simulink model "SAME5xPIM_MCLV2_MotorControl"  (R2021a)
settings: Solver=FixedStepDiscrete  StartTime=0.0  StopTime=10.0  FixedStep=5e-5  RelTol=1e-3  EnableMultiTasking=on
InitFcn:
  | % DC Voltage
  | VDC = 24;
  | 
  | % Intersective PMW
  | Vmax = VDC/2;
  | Imax = 4;
  | 
  | Ts = 1e-4;
  | 
  | 
  | % pole paires
  | p = 4;
  | 
  | % QEI
  | lines = 4*1000;
  | eleclines = lines/p;
  | inveleclines = 1/eleclines
  | gainQEIspeed = 2*pi/Ts/lines
  | 
  | % Electrical parameters
  | R=0.656; L=0.35e-3; Phif=0.0066;
  | % Mechanical parameters
  | F=1.e-05; J=1e-05; C0 = 0.01;%10;%1;
undefined symbols (not defined in the file): B27, PA08, PA09, PA10, PA11, PA12, PA13, PA16, PA17, PA18, pad0, pad1, pad2, pad3, PC16, PC17, PC18, Pin, SAME54P20A, Timer, TQFP128, wo0, wo1, wo2, wo4, wo5, wo6
libraries: MCHP_Blockset x10, simulink x8, dsparch4 x1
(part 2 of 2)

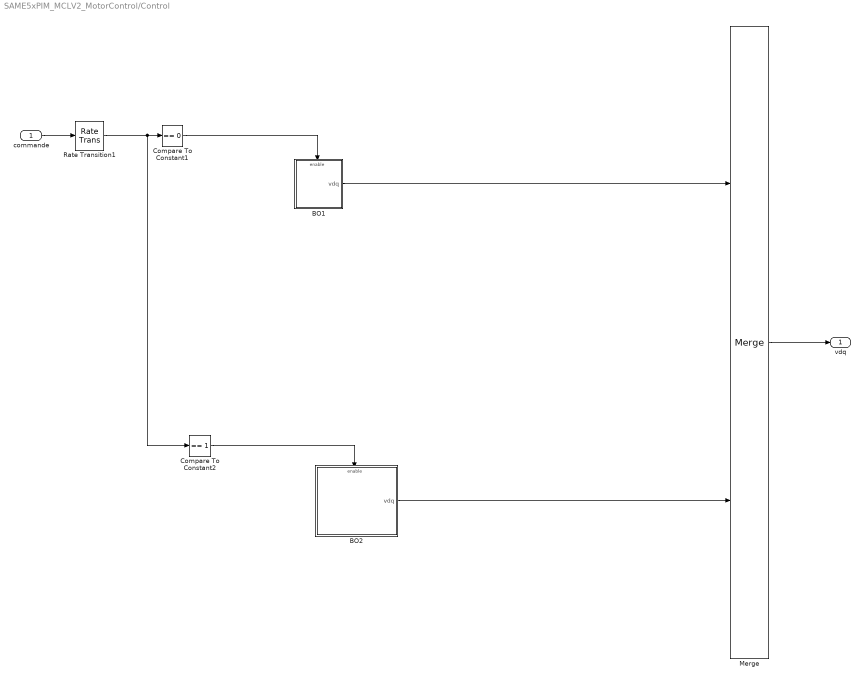
== system SAME5xPIM_MCLV2_MotorControl/Control ==
  commande : Inport
  BO1 : Subsystem
  BO2 : Subsystem
  Compare To Constant1 : simulink/Logic and Bit Operations/Compare To Constant  relop===  const=0  OutDataTypeStr=boolean
  Compare To Constant2 : simulink/Logic and Bit Operations/Compare To Constant  relop===  const=1  OutDataTypeStr=boolean
  Merge : Merge
  Rate Transition1 : RateTransition
  vdq : Outport  VectorParamsAs1DForOutWhenUnconnected=off
  wires:
  Rate Transition1/1 -> Compare To Constant1/1, Compare To Constant2/1
  Compare To Constant1/1 -> BO1/Enable
  commande/1 -> Rate Transition1/1
  Merge/1 -> vdq/1
  Compare To Constant2/1 -> BO2/Enable
  BO1/1(vdq) -> Merge/1
  BO2/1(vdq) -> Merge/2

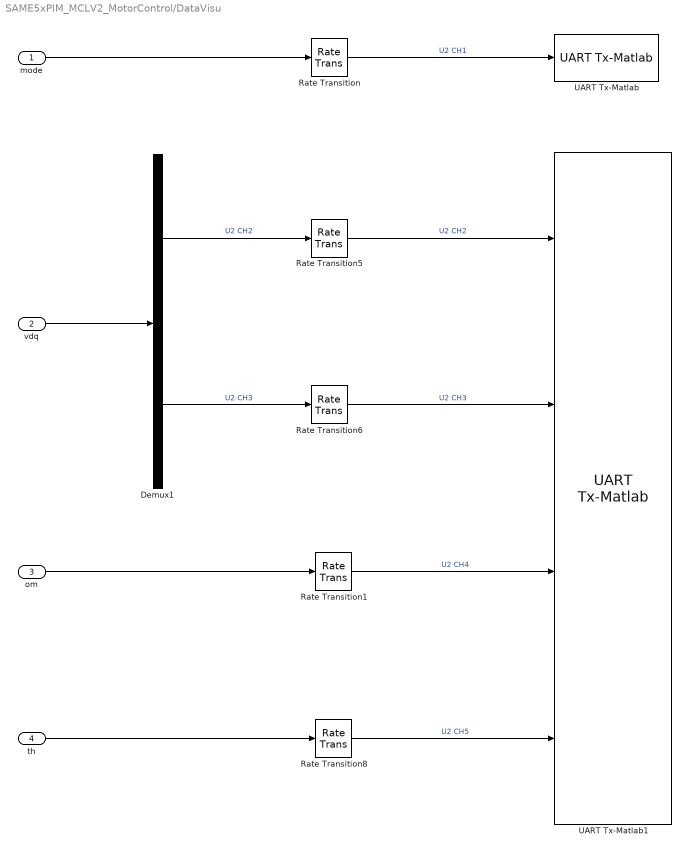
== system SAME5xPIM_MCLV2_MotorControl/DataVisu ==
  mode : Inport
  vdq : Inport  Port=2
  om : Inport  Port=3
  th : Inport  Port=4
  Demux1 : Demux  Outputs=2
  Rate Transition{,1,5..6,8} (5 alike) : RateTransition
  UART Tx-Matlab : MCHP_Blockset/BUS UART/UART Tx-Matlab  UART_REF=2  CHANNELS=[1]  AllOrNothing=off  SampleTime=.1  MCHP_MASTERLINK=SAME5xPIM_MCLV2_MotorControl/Microchip Master  MCHP_COMPILED_INFO="CompiledSampleTime= [0.10000000000000000555   0 ];CompiledInportDataTypes=[  5 ];CompiledInportDataWidth=[1];"
      settings: SourceProductName=MPLAB Device Blocks for Simulink
  UART Tx-Matlab1 : MCHP_Blockset/BUS UART/UART Tx-Matlab  UART_REF=2  CHANNELS=[2:5]  AllOrNothing=off  SampleTime=0.0005  MCHP_MASTERLINK=SAME5xPIM_MCLV2_MotorControl/Microchip Master  MCHP_COMPILED_INFO="CompiledSampleTime= [0.00050000000000000001041   0 ];CompiledInportDataTypes=[  1   1   1   1 ];CompiledInportDataWidth=[1  1  1  1];"
      settings: SourceProductName=MPLAB Device Blocks for Simulink
  wires:
  vdq/1 -> Demux1/1
  th/1 -> Rate Transition8/1
  Rate Transition5/1 -> UART Tx-Matlab1/1  "U2 CH2"
  Rate Transition8/1 -> UART Tx-Matlab1/4  "U2 CH5"
  Rate Transition1/1 -> UART Tx-Matlab1/3  "U2 CH4"
  Demux1/2 -> Rate Transition6/1  "U2 CH3"
  Rate Transition6/1 -> UART Tx-Matlab1/2  "U2 CH3"
  Demux1/1 -> Rate Transition5/1  "U2 CH2"
  om/1 -> Rate Transition1/1
  Rate Transition/1 -> UART Tx-Matlab/1  "U2 CH1"
  mode/1 -> Rate Transition/1

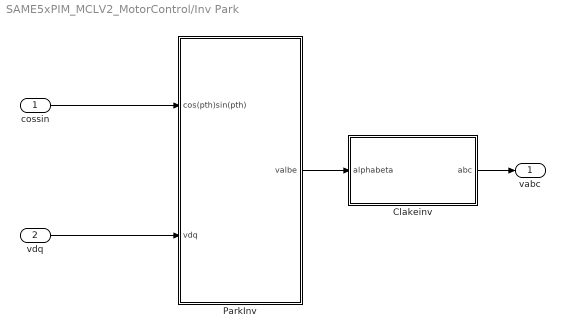
== system SAME5xPIM_MCLV2_MotorControl/Inv Park ==
  cossin : Inport
  vdq : Inport  Port=2  PortDimensions=2
  Clakeinv : Subsystem
  ParkInv : Subsystem
  vabc : Outport  VectorParamsAs1DForOutWhenUnconnected=off
  wires:
  vdq/1 -> ParkInv/2(vdq)
  cossin/1 -> ParkInv/1(cos(pth)sin(pth))
  ParkInv/1(valbe) -> Clakeinv/1(alphabeta)
  Clakeinv/1(abc) -> vabc/1

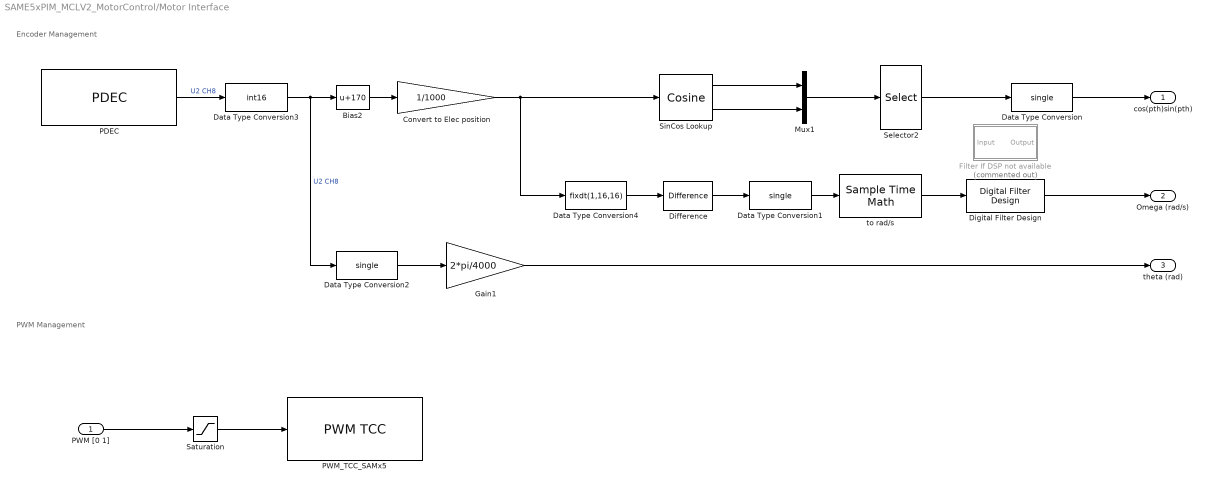
== system SAME5xPIM_MCLV2_MotorControl/Motor Interface ==
  note: Encoder Management
  note: PWM Management
  PWM [0 1] : Inport
  Bias2 : Bias  Bias=170
  Convert to Elec position : Gain  Gain=1/1000  OutDataTypeStr=fixdt(0,16,16)
  Data Type Conversion : DataTypeConversion  OutDataTypeStr=single
  Data Type Conversion1 : DataTypeConversion  OutDataTypeStr=single
  Data Type Conversion2 : DataTypeConversion  OutDataTypeStr=single
  Data Type Conversion3 : DataTypeConversion  OutDataTypeStr=int16  ConvertRealWorld=Stored Integer (SI)
  Data Type Conversion4 : DataTypeConversion  OutDataTypeStr=fixdt(1,16,16)  ConvertRealWorld=Stored Integer (SI)
  Difference : simulink/Discrete/Difference  ICPrevInput=0  OutMin=[]  OutMax=[]  OutDataType=fixdt(1, 16)  OutScaling=2^-10  DoSatur=off
  Digital Filter Design : dsparch4/Digital Filter Design  mwdsp_browser_bugfix_var=off
  Filter If DSP not available : Subsystem  Tag=FilterWizardSubSystem  Commented=on
      settings: ErrorFcn=dspFilterRealizedInBasicElemsAlgLoopErrFcnCallback
  Gain1 : Gain  Gain=2*pi/4000
  Mux1 : Mux  Inputs=2
  PDEC : MCHP_Blockset/QEI/PDEC  Mode=Quadrature Encoder  index=Reset counter  QDI0=PC16 / Pin[70]  QDI0_txt=Dynamic Options  QDI1=PC17 / Pin[71]  QDI1_txt=Dynamic Options  QDI2=PC18 / Pin[72]  QDI2_txt=Dynamic Options  maxCounterReset=-1  AutoCorrection=off  AutoCorrection_override=on  info=0  MCHP_MASTERLINK=SAME5xPIM_MCLV2_MotorControl/Microchip Master  SampleTime=1e-4  MCHP_PORT={PDEC A}{PDEC_QDI0}5:0:P80;{PDEC B}{PDEC_QDI1}5:0:P81;{PDEC index}{PDEC_QDI2}5:0:P82;  MAXPOS_INPUT=off  RESET_INPUT=off  OutputCounter=on  OutputCounter_Signed=unsigned  OutputRevolution=off  CounterRevolution_length=Counter is 13 bits ; revolution is 3 bits  OutputRevolution_Signed=unsigned  FILTER="250 (ns)  ->  freq 2 (MHz)"  FILTER_TXT="250 (ns)  ->  freq 2 (MHz)"  SWAP=off  QDI_invert_0=off  QDI_invert_1=off  QDI_invert_2=off
      settings: SourceProductName=MPLAB Device Blocks for Simulink
  PWM_TCC_SAMx5 : MCHP_Blockset/PWM IO/PWM TCC  TCCREF=TCC 0  WAVE_choice=Center aligned PWM  MaxPeriod_s=5e-5  OTMX=Default  WO0=Dynamic Options  WO0_TXT=PA08 / Pin[33] / wo0  WO1=Dynamic Options  WO1_TXT=PA09 / Pin[34] / wo1  WO2=Dynamic Options  WO2_TXT=PA10 / Pin[35] / wo2  WO3=Dynamic Options  WO3_TXT=Not Used  WO4=Dynamic Options  WO4_TXT=PA16 / Pin[66] / wo4  WO5=Dynamic Options  WO5_TXT=PA17 / Pin[67] / wo5  WO6=Dynamic Options  WO6_TXT=PA18 / Pin[68] / wo6  WO7=Dynamic Options  WO7_TXT=Not Used  info=0  evalin_ws=PWM0max=MCHP_Fun.Hex2num('40A3860000000000');PWM0max=MCHP_Fun.Hex2num('40A3860000000000');PWM0max=MCHP_Fun.Hex2num('40A3860000000000');  SampleTime=1e-4  MCHP_PORT={PWM0_H0}{TCC0_WO0}5:1:P8;{PWM0_H1}{TCC0_WO1}5:1:P9;{PWM0_H2}{TCC0_WO2}5:1:P10;{PWM0_L0}{TCC0_WO4}5:1:P16;{PWM0_L1}{TCC0_WO5}5:1:P17;{PWM0_L2}{TCC0_WO6}5:1:P18;  MCHP_MASTERLINK=SAME5xPIM_MCLV2_MotorControl/Microchip Master  INVEN_WO0=off  INVEN_WO1=off  INVEN_WO2=off  INVEN_WO3=off  INVEN_WO4=off  INVEN_WO5=off  INVEN_WO6=off  INVEN_WO7=off  SWAP_PWM0=off  SWAP_PWM1=off  SWAP_PWM2=off  SWAP_PWM3=off  POL_PWM0=off  POL_PWM1=off  POL_PWM2=off  POL_PWM3=off  POL_PWM4=off  POL_PWM5=off  InitPeriod_s=5e-5  InitDutyCycle_s=2.5e-5  InitDeadTimeH_s=0.5e-6  InitDeadTimeL_s=0.5e-6  InitOutputOverride=0  InitOutputOverride_val=0  BlockInput_VectorScalar=Vectors (grouped by function)  BlockInput_Period=Not a block input  BlockInput_DutyCycle=a Floating Point input within range [0 1]  BlockInput_DeadTime=Not a block input  BlockInput_OutputOverride=Not a block input
      settings: SourceProductName=MPLAB Device Blocks for Simulink
  Saturation : Saturate  UpperLimit=0.98  LowerLimit=0.02  LinearizeAsGain=off  OutDataTypeStr=double
  Selector2 : Selector  InputPortWidth=2  IndexOptions=Index vector (dialog)  Indices=[2 1]  OutputSizes=1
  SinCos Lookup : simulink/Lookup Tables/Cosine  Formula=sin(2*pi*u) and cos(2*pi*u)  NumDataPoints=(2^12)+1  OutputWordLength=16  InternalRulePriority=Precision
      settings: SourceProductBaseCode=SL
  to rad/s : SampleTimeMath  TsampMathOp=/  weightValue=(4)/(2*pi)
  cos(pth)sin(pth) : Outport  VectorParamsAs1DForOutWhenUnconnected=off
  Omega (rad/s) : Outport  Port=2  PortDimensions=1  VectorParamsAs1DForOutWhenUnconnected=off
  theta (rad) : Outport  Port=3  VectorParamsAs1DForOutWhenUnconnected=off
  wires:
  Saturation/1 -> PWM_TCC_SAMx5/1
  PWM [0 1]/1 -> Saturation/1
  Convert to Elec position/1 -> Data Type Conversion4/1, SinCos Lookup/1
  to rad/s/1 -> Digital Filter Design/1
  Bias2/1 -> Convert to Elec position/1
  PDEC/1 -> Data Type Conversion3/1  "U2 CH8"
  Digital Filter Design/1 -> Omega (rad/s)/1
  Data Type Conversion/1 -> cos(pth)sin(pth)/1
  Mux1/1 -> Selector2/1
  Selector2/1 -> Data Type Conversion/1
  SinCos Lookup/2 -> Mux1/2
  SinCos Lookup/1 -> Mux1/1
  Data Type Conversion3/1 -> Data Type Conversion2/1, Bias2/1  "U2 CH8"
  Data Type Conversion2/1 -> Gain1/1
  Gain1/1 -> theta (rad)/1
  Difference/1 -> Data Type Conversion1/1
  Data Type Conversion4/1 -> Difference/1
  Data Type Conversion1/1 -> to rad/s/1

== system SAME5xPIM_MCLV2_MotorControl/PWM ==
  vabc : Inport
  50% average duty-cycle : Bias  Bias=0.5
  Gain : Gain  Gain=1/VDC  OutDataTypeStr=double
  PWM [0 1] : Outport  VectorParamsAs1DForOutWhenUnconnected=off
  wires:
  vabc/1 -> Gain/1
  50% average duty-cycle/1 -> PWM [0 1]/1
  Gain/1 -> 50% average duty-cycle/1

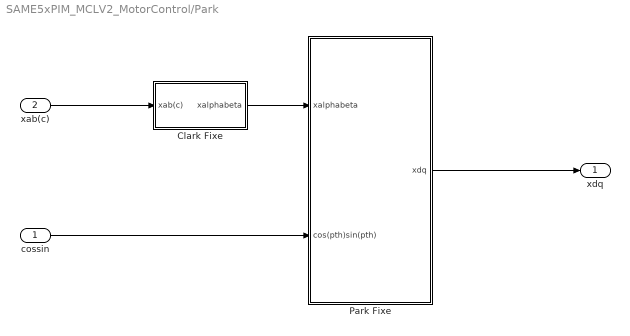
== system SAME5xPIM_MCLV2_MotorControl/Park  ==
  cossin : Inport
  xab(c) : Inport  Port=2
  Clark Fixe : Subsystem
  Park Fixe : Subsystem
  xdq : Outport  VectorParamsAs1DForOutWhenUnconnected=off
  wires:
  Clark Fixe/1(xalphabeta) -> Park Fixe/1(xalphabeta)
  xab(c)/1 -> Clark Fixe/1(xab(c))
  cossin/1 -> Park Fixe/2(cos(pth)sin(pth))
  Park Fixe/1(xdq) -> xdq/1

== system SAME5xPIM_MCLV2_MotorControl/Selector ==
  BTN_S2 : MCHP_Blockset/Digital IO/Digital Input  PORT=Dynamic Options  PORT_TXT="D   [ 0  1  8  9  10  11  12  20  21 ]"  PIN=9  PACK=off  SIMULTANEOUS=off  ORDERING=None  SampleTime=.1  MCHP_PORT={Digital In}{DIN}2:0:D9;  MCHP_MASTERLINK=SAME5xPIM_MCLV2_MotorControl/Microchip Master
      settings: SourceProductName=MPLAB Device Blocks for Simulink
  Toggle (4 states)1 : Subsystem
  Mode : Outport  VectorParamsAs1DForOutWhenUnconnected=off
  tag scope: mode=global
  wires:
  BTN_S2/1 -> Toggle (4 states)1/1(In1)
  Toggle (4 states)1/1(Mode) -> [mode], Mode/1

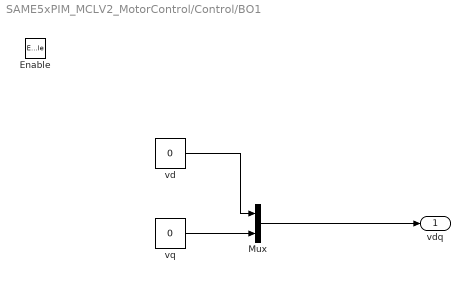
== system SAME5xPIM_MCLV2_MotorControl/Control/BO1 ==
  Enable : EnablePort
  Mux : Mux  Inputs=2
  vd : Constant  Value=0  OutMin=[-12]  OutMax=[12]  OutDataTypeStr=single
  vq : Constant  Value=0  OutMin=[-12]  OutMax=[12]  OutDataTypeStr=single
  vdq : Outport  VectorParamsAs1DForOutWhenUnconnected=off
  wires:
  vd/1 -> Mux/1
  Mux/1 -> vdq/1
  vq/1 -> Mux/2

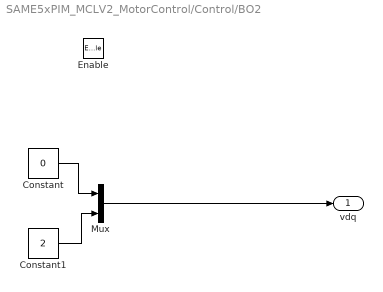
== system SAME5xPIM_MCLV2_MotorControl/Control/BO2 ==
  Enable : EnablePort
  Constant : Constant  Value=0  OutDataTypeStr=single
  Constant1 : Constant  Value=2  OutDataTypeStr=single
  Mux : Mux  Inputs=2
  vdq : Outport  VectorParamsAs1DForOutWhenUnconnected=off
  wires:
  Constant1/1 -> Mux/2
  Constant/1 -> Mux/1
  Mux/1 -> vdq/1

== system SAME5xPIM_MCLV2_MotorControl/Inv Park/Clakeinv ==
  alphabeta : Inport
  Clarke1 : Product  Multiplication=Matrix(*)  RndMeth=Simplest  OutDataTypeStr=Inherit: Same as first input
  Constant Magnitude : Constant  Value=[1 0 ; -1/2 sqrt(3)/2 ;-1/2 -sqrt(3)/2]'  OutDataTypeStr=Inherit: Inherit via back propagation  SampleTime=-1
  Math Function : Math  Operator=transpose  SignedPower=on  SaturateOnIntegerOverflow=on
  abc : Outport  VectorParamsAs1DForOutWhenUnconnected=off
  wires:
  alphabeta/1 -> Math Function/1
  Constant Magnitude/1 -> Clarke1/2
  Math Function/1 -> Clarke1/1
  Clarke1/1 -> abc/1

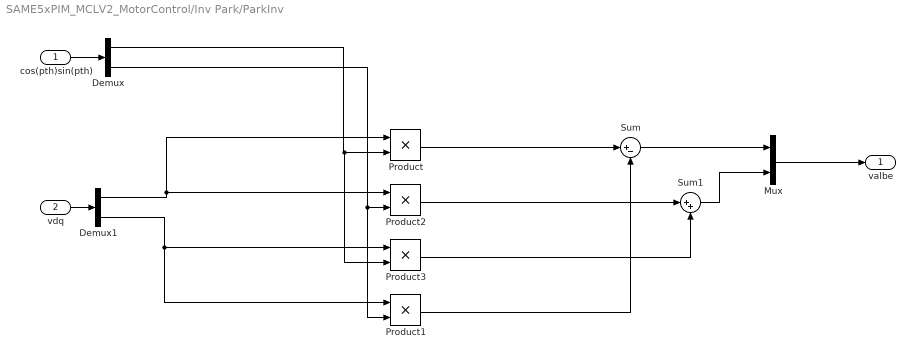
== system SAME5xPIM_MCLV2_MotorControl/Inv Park/ParkInv ==
  cos(pth)sin(pth) : Inport
  vdq : Inport  Port=2
  Demux : Demux  Outputs=2
  Demux1 : Demux  Outputs=2
  Mux : Mux  Inputs=2
  Product{,1..3} (4 alike) : Product
  Sum : Sum  Inputs=|+-
  Sum1 : Sum  Inputs=|++
  valbe : Outport  VectorParamsAs1DForOutWhenUnconnected=off
  wires:
  vdq/1 -> Demux1/1
  cos(pth)sin(pth)/1 -> Demux/1
  Sum/1 -> Mux/1
  Demux1/1 -> Product2/1, Product/1
  Demux1/2 -> Product3/1, Product1/1
  Sum1/1 -> Mux/2
  Product1/1 -> Sum/2
  Product/1 -> Sum/1
  Demux/1 -> Product3/2, Product/2
  Demux/2 -> Product2/2, Product1/2
  Mux/1 -> valbe/1
  Product2/1 -> Sum1/1
  Product3/1 -> Sum1/2

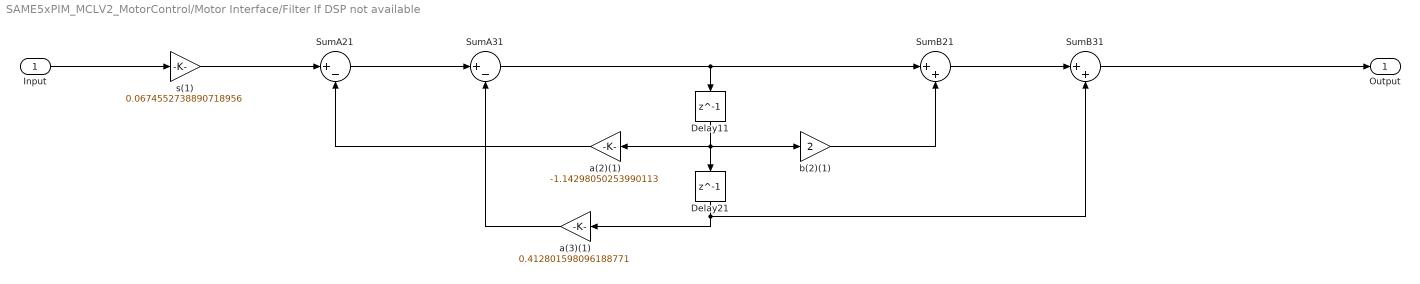
== system SAME5xPIM_MCLV2_MotorControl/Motor Interface/Filter If DSP not available ==
  Input : Inport
  Delay11 : Delay  DelayLength=1  InitialCondition=0
  Delay21 : Delay  DelayLength=1  InitialCondition=0
  SumA21 : Sum  Inputs=|+-  RndMeth=Nearest  SaturateOnIntegerOverflow=on  OutDataTypeStr=Inherit: Same as first input
  SumA31 : Sum  Inputs=|+-  RndMeth=Nearest  SaturateOnIntegerOverflow=on  OutDataTypeStr=Inherit: Same as first input
  SumB21 : Sum  Inputs=|++  RndMeth=Nearest  SaturateOnIntegerOverflow=on  OutDataTypeStr=Inherit: Same as first input
  SumB31 : Sum  Inputs=|++  RndMeth=Nearest  SaturateOnIntegerOverflow=on  OutDataTypeStr=Inherit: Same as first input
  a(2)(1) : Gain  Gain=-1.14298050253990113  ParamDataTypeStr=double  RndMeth=Nearest  SaturateOnIntegerOverflow=on  OutDataTypeStr=Inherit: Same as input
  a(3)(1) : Gain  Gain=0.412801598096188771  ParamDataTypeStr=double  RndMeth=Nearest  SaturateOnIntegerOverflow=on  OutDataTypeStr=Inherit: Same as input
  b(2)(1) : Gain  Gain=2  ParamDataTypeStr=double  RndMeth=Nearest  SaturateOnIntegerOverflow=on  OutDataTypeStr=Inherit: Same as input
  s(1) : Gain  Gain=0.0674552738890718956  ParamDataTypeStr=double  RndMeth=Nearest  SaturateOnIntegerOverflow=on  OutDataTypeStr=Inherit: Same as input
  Output : Outport
  wires:
  Delay21/1 -> SumB31/2, a(3)(1)/1
  a(3)(1)/1 -> SumA31/2
  b(2)(1)/1 -> SumB21/2
  Delay11/1 -> Delay21/1, b(2)(1)/1, a(2)(1)/1
  a(2)(1)/1 -> SumA21/2
  SumB31/1 -> Output/1
  SumB21/1 -> SumB31/1
  SumA31/1 -> Delay11/1, SumB21/1
  SumA21/1 -> SumA31/1
  s(1)/1 -> SumA21/1
  Input/1 -> s(1)/1

== system SAME5xPIM_MCLV2_MotorControl/Park /Clark Fixe ==
  note: Input is a vector of 3 elements, 3rd element is not beeing used
  note: k = 2/3 : invariant Magnitude
  xab(c) : Inport
  Clarke1 : Product  Multiplication=Matrix(*)  OutDataTypeStr=single  RndMeth=Convergent  SaturateOnIntegerOverflow=on
  Constant Magnitude : Constant  Value=[1 0 ; 1/sqrt(3) 2/sqrt(3) ];  OutDataTypeStr=single
  xalphabeta : Outport  VectorParamsAs1DForOutWhenUnconnected=off
  wires:
  Clarke1/1 -> xalphabeta/1
  Constant Magnitude/1 -> Clarke1/1
  xab(c)/1 -> Clarke1/2

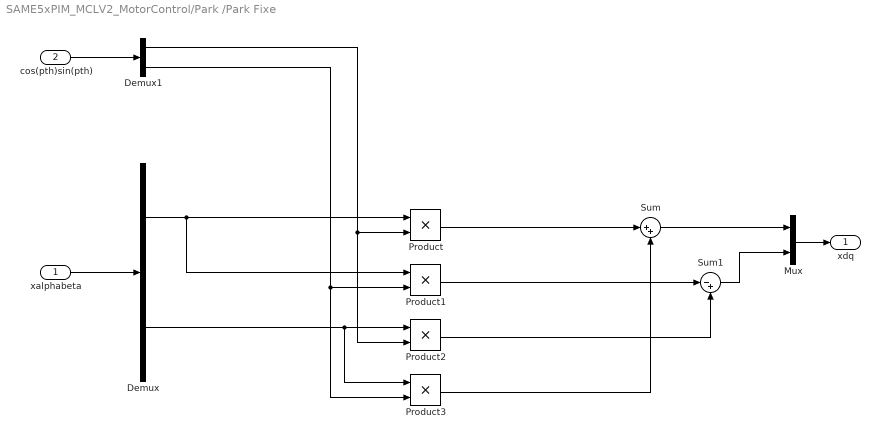
== system SAME5xPIM_MCLV2_MotorControl/Park /Park Fixe ==
  xalphabeta : Inport
  cos(pth)sin(pth) : Inport  Port=2
  Demux : Demux  Outputs=2
  Demux1 : Demux  Outputs=2
  Mux : Mux  Inputs=2
  Product{,1..3} (4 alike) : Product
  Sum : Sum  Inputs=|++  SaturateOnIntegerOverflow=on
  Sum1 : Sum  Inputs=|-+  SaturateOnIntegerOverflow=on
  xdq : Outport  VectorParamsAs1DForOutWhenUnconnected=off
  wires:
  cos(pth)sin(pth)/1 -> Demux1/1
  Product2/1 -> Sum1/2
  Product1/1 -> Sum1/1
  Demux1/2 -> Product3/2, Product1/2
  Demux1/1 -> Product2/2, Product/2
  Product/1 -> Sum/1
  Product3/1 -> Sum/2
  Sum1/1 -> Mux/2
  Demux/2 -> Product3/1, Product2/1
  Demux/1 -> Product1/1, Product/1
  Sum/1 -> Mux/1
  Mux/1 -> xdq/1
  xalphabeta/1 -> Demux/1

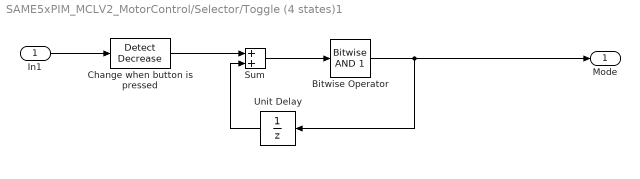
== system SAME5xPIM_MCLV2_MotorControl/Selector/Toggle (4 states)1 ==
  In1 : Inport
  Bitwise Operator : simulink/Logic and Bit Operations/Bitwise Operator  logicop=AND  UseBitMask=on  BitMask=1  BitMaskRealWorld=Stored Integer
  Change when button is pressed : simulink/Logic and Bit Operations/Detect Decrease  vinit=0.0  OutDataTypeStr=uint8
  Sum : Sum  AccumDataTypeStr=uint16  OutDataTypeStr=uint16
  Unit Delay : UnitDelay  SampleTime=-1  HasFrameUpgradeWarning=on
  Mode : Outport  VectorParamsAs1DForOutWhenUnconnected=off
  wires:
  Change when button is pressed/1 -> Sum/1
  Bitwise Operator/1 -> Mode/1, Unit Delay/1
  Unit Delay/1 -> Sum/2
  Sum/1 -> Bitwise Operator/1
  In1/1 -> Change when button is pressed/1
